simulink model "Copy_of_Kalman"  (R2021a)
settings: Solver=VariableStepAuto  StartTime=0.0  StopTime=10.0  RelTol=1e-3
values from neighbouring files (symbols this model uses):
  ff = 1.1    [Analyze.m]
  ground_alt = mean(z_hypsometric(ground_pressure))    [Analyze.m]
undefined symbols (not defined in the file or in its folder): Discrete, Time
libraries: ctrlSharedLib x5
settings Model: Creator=jtc12  LastModifiedBy=Willi

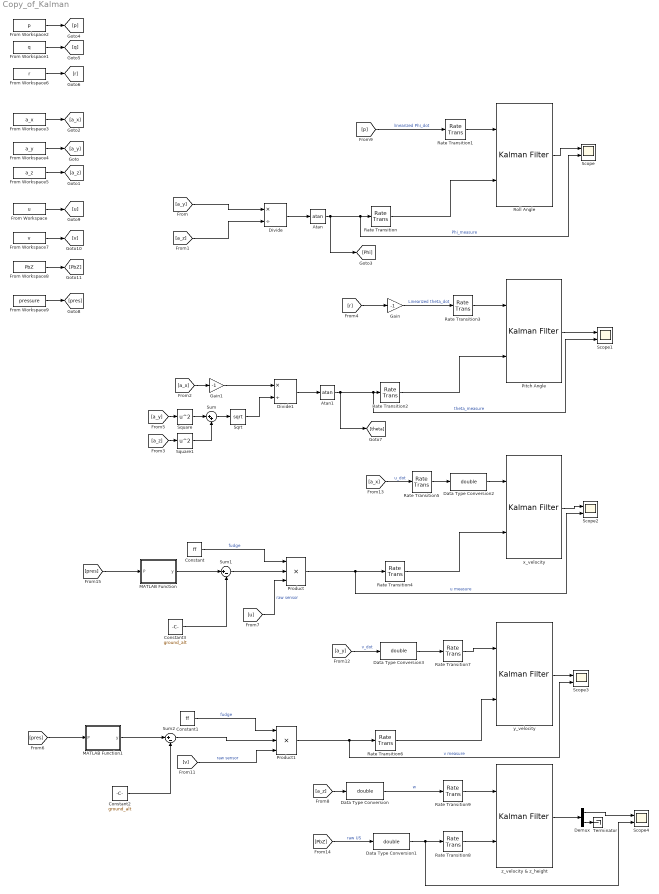
== system Copy_of_Kalman ==
  Atan : Trigonometry  Operator=atan
  Atan1 : Trigonometry  Operator=atan
  Constant : Constant  Value=ff
  Constant1 : Constant  Value=ff
  Constant2 : Constant  Value=ground_alt
  Constant3 : Constant  Value=ground_alt
  Data Type Conversion{,1..3} (4 alike) : DataTypeConversion  OutDataTypeStr=double
  Demux : Demux  Outputs=2
  Divide : Product  Inputs=*/
  Divide1 : Product  Inputs=*/
  From Workspace : FromWorkspace  VariableName=u
  From Workspace1 : FromWorkspace  VariableName=q
  From Workspace2 : FromWorkspace  VariableName=p
  From Workspace3 : FromWorkspace  VariableName=a_x
  From Workspace4 : FromWorkspace  VariableName=a_y
  From Workspace5 : FromWorkspace  VariableName=a_z
  From Workspace6 : FromWorkspace  VariableName=r
  From Workspace7 : FromWorkspace  VariableName=v
  From Workspace8 : FromWorkspace  VariableName=PbZ
  From Workspace9 : FromWorkspace  VariableName=pressure
  Gain : Gain  Gain=-1
  Gain1 : Gain  Gain=-1
  MATLAB Function : MATLAB Function  TreatAsAtomicUnit=on
  MATLAB Function1 : MATLAB Function  TreatAsAtomicUnit=on
  Pitch Angle : ctrlSharedLib/Kalman Filter  TimeDomain=Discrete-Time  UseCurrentEstimator=on  ModelSource=Individual A, B, C, D matrices  ModelSourceVariable=ss(0.95,1,1,0,1)  A=[1]  B=[1/200]  C=[1]  D=0  NumberOfStates=1  NumberOfInputs=1  NumberOfOutputs=1  InitialEstimateSource=Dialog  X0=0  P0=10  UseK=off  UseGH=off  NumberOfProcessNoiseInputs=1  G=1  TimeInvariantG=on  H=0  TimeInvariantH=on  Q=.0085/200  TimeInvariantQ=on  R=.0066  TimeInvariantR=on  N=0  TimeInvariantN=on  AddInputPort=on  AddEnablePort=off  OutputEstimatedY=off  OutputP=off  Ts=-1
  Product : Product  Inputs=3
  Product1 : Product  Inputs=3
  Rate Transition{,1..9} (10 alike) : RateTransition  OutPortSampleTime=1/200
  Roll Angle : ctrlSharedLib/Kalman Filter  TimeDomain=Discrete-Time  UseCurrentEstimator=on  ModelSource=Individual A, B, C, D matrices  ModelSourceVariable=ss(0.95,1,1,0,1)  A=[1]  B=[1/200]  C=[1]  D=0  NumberOfStates=1  NumberOfInputs=1  NumberOfOutputs=1  InitialEstimateSource=Dialog  X0=0  P0=10  UseK=off  UseGH=off  NumberOfProcessNoiseInputs=1  G=1  TimeInvariantG=on  H=0  TimeInvariantH=on  Q=.0133/200  TimeInvariantQ=on  R=.0101  TimeInvariantR=on  N=0  TimeInvariantN=on  AddInputPort=on  AddEnablePort=off  OutputEstimatedY=off  OutputP=off  Ts=-1
  Scope{,1..4} (5 alike) : Scope  NumInputPorts=2
  Sqrt : Sqrt  SaturateOnIntegerOverflow=on
  Square : Math  Operator=square  SaturateOnIntegerOverflow=on
  Square1 : Math  Operator=square  SaturateOnIntegerOverflow=on
  Sum : Sum  Inputs=|++
  Sum1 : Sum  Inputs=|+-
  Sum2 : Sum  Inputs=|+-
  Terminator : Terminator
  x_velocity : ctrlSharedLib/Kalman Filter  TimeDomain=Discrete-Time  UseCurrentEstimator=on  ModelSource=Individual A, B, C, D matrices  ModelSourceVariable=ss(0.95,1,1,0,1)  A=[1 ]  B=[1/200]  C=[1]  D=0  NumberOfStates=1  NumberOfInputs=1  NumberOfOutputs=1  InitialEstimateSource=Dialog  X0=0  P0=10  UseK=off  UseGH=off  NumberOfProcessNoiseInputs=1  G=1  TimeInvariantG=on  H=0  TimeInvariantH=on  Q=.0059/200  TimeInvariantQ=on  R=2.67  TimeInvariantR=on  N=0  TimeInvariantN=on  AddInputPort=on  AddEnablePort=off  OutputEstimatedY=off  OutputP=off  Ts=-1
  y_velocity : ctrlSharedLib/Kalman Filter  TimeDomain=Discrete-Time  UseCurrentEstimator=on  ModelSource=Individual A, B, C, D matrices  ModelSourceVariable=ss(0.95,1,1,0,1)  A=[1]  B=[1/200]  C=[1 ]  D=0  NumberOfStates=1  NumberOfInputs=1  NumberOfOutputs=1  InitialEstimateSource=Dialog  X0=0  P0=10  UseK=off  UseGH=off  NumberOfProcessNoiseInputs=1  G=1  TimeInvariantG=on  H=0  TimeInvariantH=on  Q=.0087/200  TimeInvariantQ=on  R=2.5  TimeInvariantR=on  N=0  TimeInvariantN=on  AddInputPort=on  AddEnablePort=off  OutputEstimatedY=off  OutputP=off  Ts=-1
  z_velocity & z_height : ctrlSharedLib/Kalman Filter  TimeDomain=Discrete-Time  UseCurrentEstimator=on  ModelSource=Individual A, B, C, D matrices  ModelSourceVariable=ss(0.95,1,1,0,1)  A=[1 1/200; 0 1;]  B=[1/2*(1/200)^2; 1/200]  C=[1 0]  D=0  NumberOfStates=1  NumberOfInputs=1  NumberOfOutputs=1  InitialEstimateSource=Dialog  X0=0  P0=10  UseK=off  UseGH=off  NumberOfProcessNoiseInputs=1  G=1  TimeInvariantG=on  H=0  TimeInvariantH=on  Q=1  TimeInvariantQ=on  R=1  TimeInvariantR=on  N=0  TimeInvariantN=on  AddInputPort=on  AddEnablePort=off  OutputEstimatedY=off  OutputP=off  Ts=-1
  wires:
  [a_y] -> Divide/1
  [a_z] -> Divide/2
  Divide/1 -> Atan/1
  From Workspace3/1 -> [a_x]
  From Workspace4/1 -> [a_y]
  From Workspace5/1 -> [a_z]
  Atan/1 -> [Phi], Scope/2, Rate Transition/1  "Phi_measure"
  Rate Transition/1 -> Roll Angle/2
  From Workspace2/1 -> [p]
  From Workspace1/1 -> [q]
  From Workspace6/1 -> [r]
  Rate Transition1/1 -> Roll Angle/1
  [p] -> Rate Transition1/1  "linearized Phi_dot"
  Atan1/1 -> [theta], Scope1/2, Rate Transition2/1  "theta_measure"
  Rate Transition2/1 -> Pitch Angle/2
  Rate Transition3/1 -> Pitch Angle/1
  Pitch Angle/1 -> Scope1/1
  Divide1/1 -> Atan1/1
  [r] -> Gain/1
  Gain/1 -> Rate Transition3/1  "Linearized theta_dot"
  [a_x] -> Gain1/1
  Gain1/1 -> Divide1/1
  [a_y] -> Square/1
  [a_z] -> Square1/1
  Square/1 -> Sum/1
  Square1/1 -> Sum/2
  Sum/1 -> Sqrt/1
  Sqrt/1 -> Divide1/2
  x_velocity/1 -> Scope2/1
  Rate Transition4/1 -> x_velocity/2
  From Workspace/1 -> [u]
  From Workspace7/1 -> [v]
  From Workspace8/1 -> [PbZ]
  Constant/1 -> Product/1  "fudge"
  [u] -> Product/3  "raw sensor"
  Product/1 -> Scope2/2, Rate Transition4/1  "u measure"
  Rate Transition7/1 -> y_velocity/1
  y_velocity/1 -> Scope3/1
  Product1/1 -> Scope3/2, Rate Transition6/1  "v measure"
  Rate Transition6/1 -> y_velocity/2
  Constant1/1 -> Product1/1  "fudge"
  [v] -> Product1/3  "raw sensor"
  [a_x] -> Rate Transition5/1  "u_dot"
  Rate Transition8/1 -> z_velocity & z_height/2
  Rate Transition9/1 -> z_velocity & z_height/1
  Data Type Conversion/1 -> Rate Transition9/1  "w"
  [a_z] -> Data Type Conversion/1
  Data Type Conversion1/1 -> Scope4/2, Rate Transition8/1
  [PbZ] -> Data Type Conversion1/1  "raw US"
  Rate Transition5/1 -> Data Type Conversion2/1
  Data Type Conversion2/1 -> x_velocity/1
  [a_y] -> Data Type Conversion3/1  "v_dot"
  Data Type Conversion3/1 -> Rate Transition7/1
  Roll Angle/1 -> Scope/1
  From Workspace9/1 -> [pres]
  [pres] -> MATLAB Function/1(P)
  Sum2/1 -> Product1/2
  Sum1/1 -> Product/2
  MATLAB Function/1(y) -> Sum1/1
  Constant3/1 -> Sum1/2
  Constant2/1 -> Sum2/2
  MATLAB Function1/1(y) -> Sum2/1
  [pres] -> MATLAB Function1/1(P)
  Demux/2 -> Terminator/1
  z_velocity & z_height/1 -> Demux/1
  Demux/1 -> Scope4/1

== matlab function Copy_of_Kalman/MATLAB Function ==
  data: P input; y output
function y = z_pres(P)
g = 9.8; % acceleration due to gravity m/s^2
M = 0.0289644; % molar mass of air in kg/mol
R = 8.31432; % universal gas constant Nm/mol/k
p0 = 101325; % Pa standard pressure

T =288.15;  % Assumed temperature in kelvin
K =-g*M/R/T;
z_hypsometric = 1/K.*log(P./p0);
y = z_hypsometric;

== matlab function Copy_of_Kalman/MATLAB Function1 ==
  data: P input; y output
function y = z_pres(P)
g = 9.8; % acceleration due to gravity m/s^2
M = 0.0289644; % molar mass of air in kg/mol
R = 8.31432; % universal gas constant Nm/mol/k
p0 = 101325; % Pa standard pressure

T =288.15;  % Assumed temperature in kelvin
K =-g*M/R/T;
z_hypsometric = 1/K.*log(P./p0);
y = z_hypsometric;
